simulink model "Simulation_Fahrmodell_v4_straight_line_v1"  (R2023b)
settings: Solver=ode14x  StartTime=0.0  StopTime=500  FixedStep=0.005  RelTol=1e-3
undefined symbols (not defined in the file): bat, cp, cp_Zelle_JpkgK, gb, Ice_derfacLoadDecrease_MAP, Ice_derfacLoadIncrease_MAP, Ice_n_axis, Ice_relLoadMax_CUR_n, Ice_relLoadMax_CUR_val, Ice_rl_axis_norm, P4, P4_DM, pt, seconds, SKO_STREET_CHAL, SKO_WHEEL_TYP_CHAL, slip_pacejka, T_init_degC, Track, TT_sliced, use_turbo_model, v_Fzg_init_kmph, veh
libraries: nesl_utility x15, fl_lib x9, simulink x4
(part 6 of 7)

== system Simulation_Fahrmodell_v4_straight_line_v1/Vehicle Dynamics Model /Drivetrain/Primary and Secondary Axle Powertrain Selector/Primary Axle Powertrain Selector/Electric Drive/Variant Subsystem/EV Single Motor/Battery and Operating Strategy Limitation (Drive)/Discharge Limit ==
  Torque_Drive_In : Inport
  Gain2 : Gain  Gain=100
  MATLAB Function : MATLAB Function  TreatAsAtomicUnit=on
  Recuperation Limit2 : Constant  Value=bat.SOC_Bat_Discharge_Limit
  Torque_Drive_Out : Outport
  wires:
  Torque_Drive_In/1 -> MATLAB Function/1(Torque_In)
  Recuperation Limit2/1 -> Gain2/1
  MATLAB Function/1(Torque_Out) -> Torque_Drive_Out/1
  [SOC] -> MATLAB Function/2(SOC)
  Gain2/1 -> MATLAB Function/3(Discharge_Limit)

== system Simulation_Fahrmodell_v4_straight_line_v1/Vehicle Dynamics Model /Drivetrain/Primary and Secondary Axle Powertrain Selector/Primary Axle Powertrain Selector/Electric Drive/Variant Subsystem/EV Single Motor/Battery and Operating Strategy Limitation (Recuperation)/Begrenzung BAT + Betriebsstrategie EM EV, Reku2 ==
  n_Upmin IN : Inport
  M_Nm : Inport  Port=2
  P_mech_max_kW : Inport  Port=3
  Max1 : MinMax  Function=max  Inputs=2
  "P_kW -> M_Nm" : Subsystem
  n_Upmin OUT : Outport
  M_begr_Nm : Outport  Port=2
  wires:
  M_Nm/1 -> Max1/1
  Max1/1 -> M_begr_Nm/1
  "P_kW -> M_Nm"/1(Out1) -> Max1/2  "M_mech_max_Nm"
  n_Upmin IN/1 -> "P_kW -> M_Nm"/2(In2), n_Upmin OUT/1
  P_mech_max_kW/1 -> "P_kW -> M_Nm"/1(P_kW)  "P_kW"

== system Simulation_Fahrmodell_v4_straight_line_v1/Vehicle Dynamics Model /Drivetrain/Primary and Secondary Axle Powertrain Selector/Primary Axle Powertrain Selector/Electric Drive/Variant Subsystem/EV Single Motor/Battery and Operating Strategy Limitation (Recuperation)/Recuperation Limit ==
  Torque_Recu_In : Inport
  Constant : Constant  Value=0
  Gain5 : Gain  Gain=100
  Recuperation Limit : Constant  Value=bat.SOC_Recup_Limit
  Relational Operator2 : RelationalOperator  Operator=<  OutDataTypeStr=boolean  RndMeth=Simplest  InputSameDT=off
  Switch2 : Switch  Criteria=u2 > Threshold  SaturateOnIntegerOverflow=off  InputSameDT=off
  Torque_Recu_Out : Outport
  wires:
  Constant/1 -> Switch2/3
  [SOC] -> Relational Operator2/1
  Recuperation Limit/1 -> Gain5/1
  Relational Operator2/1 -> Switch2/2
  Torque_Recu_In/1 -> Switch2/1
  Switch2/1 -> Torque_Recu_Out/1
  Gain5/1 -> Relational Operator2/2

== system Simulation_Fahrmodell_v4_straight_line_v1/Vehicle Dynamics Model /Drivetrain/Primary and Secondary Axle Powertrain Selector/Primary Axle Powertrain Selector/Hybrid Drive/P0/P0 Motor/Battery and Operating Strategy Limitation (Recuperation)/Begrenzung BAT + Betriebsstrategie EM P2, Reku1 ==
  n_Upmin IN : Inport
  M_Nm : Inport  Port=2
  P_mech_max_kW : Inport  Port=3
  Max1 : MinMax  Function=max  Inputs=2
  "P_kW -> M_Nm" : Subsystem
  n_Upmin OUT : Outport
  M_begr_Nm : Outport  Port=2
  wires:
  M_Nm/1 -> Max1/1
  Max1/1 -> M_begr_Nm/1
  "P_kW -> M_Nm"/1(Out1) -> Max1/2  "M_mech_max_Nm"
  n_Upmin IN/1 -> "P_kW -> M_Nm"/2(In2), n_Upmin OUT/1
  P_mech_max_kW/1 -> "P_kW -> M_Nm"/1(P_kW)  "P_kW"

== system Simulation_Fahrmodell_v4_straight_line_v1/Vehicle Dynamics Model /Drivetrain/Primary and Secondary Axle Powertrain Selector/Primary Axle Powertrain Selector/Hybrid Drive/P0/P0 Motor/Battery and Operating Strategy Limitation (Recuperation)/Recuperation Limit1 ==
  Torque_Recu_In : Inport
  Constant : Constant  Value=0
  Gain5 : Gain  Gain=100
  Recuperation Limit : Constant  Value=bat.SOC_Recup_Limit
  Relational Operator2 : RelationalOperator  Operator=<  OutDataTypeStr=boolean  RndMeth=Simplest  InputSameDT=off
  Switch2 : Switch  Criteria=u2 > Threshold  SaturateOnIntegerOverflow=off  InputSameDT=off
  Torque_Recu_Out : Outport
  wires:
  Constant/1 -> Switch2/3
  [SOC] -> Relational Operator2/1
  Recuperation Limit/1 -> Gain5/1
  Relational Operator2/1 -> Switch2/2
  Torque_Recu_In/1 -> Switch2/1
  Switch2/1 -> Torque_Recu_Out/1
  Gain5/1 -> Relational Operator2/2

== system Simulation_Fahrmodell_v4_straight_line_v1/Vehicle Dynamics Model /Drivetrain/Primary and Secondary Axle Powertrain Selector/Primary Axle Powertrain Selector/Hybrid Drive/P0/P0 Motor/SubsysteBattery and Operating Strategy Limitation (Drive)m/Begrenzung BAT + Betriebsstrategie EM P2, Fahren1 ==
  n_Upmin IN : Inport
  M_Nm : Inport  Port=2
  P_mech_max_kW : Inport  Port=3
  Max1 : MinMax  Inputs=2
  "P_kW -> M_Nm" : Subsystem
  n_Upmin OUT : Outport
  M_begr_Nm : Outport  Port=2
  wires:
  M_Nm/1 -> Max1/1
  Max1/1 -> M_begr_Nm/1
  "P_kW -> M_Nm"/1(Out1) -> Max1/2  "M_mech_max_Nm"
  n_Upmin IN/1 -> "P_kW -> M_Nm"/2(In2), n_Upmin OUT/1
  P_mech_max_kW/1 -> "P_kW -> M_Nm"/1(P_kW)  "P_kW"

== system Simulation_Fahrmodell_v4_straight_line_v1/Vehicle Dynamics Model /Drivetrain/Primary and Secondary Axle Powertrain Selector/Primary Axle Powertrain Selector/Hybrid Drive/P0/P0 Motor/SubsysteBattery and Operating Strategy Limitation (Drive)m/Discharge Limit ==
  Torque_Drive_In : Inport
  Gain2 : Gain  Gain=100
  MATLAB Function : MATLAB Function  TreatAsAtomicUnit=on
  Recuperation Limit2 : Constant  Value=bat.SOC_Bat_Discharge_Limit
  Torque_Drive_Out : Outport
  wires:
  Torque_Drive_In/1 -> MATLAB Function/1(Torque_In)
  Recuperation Limit2/1 -> Gain2/1
  MATLAB Function/1(Torque_Out) -> Torque_Drive_Out/1
  [SOC] -> MATLAB Function/2(SOC)
  Gain2/1 -> MATLAB Function/3(Discharge_Limit)

== system Simulation_Fahrmodell_v4_straight_line_v1/Vehicle Dynamics Model /Drivetrain/Primary and Secondary Axle Powertrain Selector/Primary Axle Powertrain Selector/Hybrid Drive/P2/P2 Motor/Battery and Operating Strategy Limitation (Drive)/Begrenzung BAT + Betriebsstrategie EM P2, Fahren1 ==
  n_Upmin IN : Inport
  M_Nm : Inport  Port=2
  P_mech_max_kW : Inport  Port=3
  Max1 : MinMax  Inputs=2
  "P_kW -> M_Nm" : Subsystem
  n_Upmin OUT : Outport
  M_begr_Nm : Outport  Port=2
  wires:
  M_Nm/1 -> Max1/1
  Max1/1 -> M_begr_Nm/1
  "P_kW -> M_Nm"/1(Out1) -> Max1/2  "M_mech_max_Nm"
  n_Upmin IN/1 -> "P_kW -> M_Nm"/2(In2), n_Upmin OUT/1
  P_mech_max_kW/1 -> "P_kW -> M_Nm"/1(P_kW)  "P_kW"

== system Simulation_Fahrmodell_v4_straight_line_v1/Vehicle Dynamics Model /Drivetrain/Primary and Secondary Axle Powertrain Selector/Primary Axle Powertrain Selector/Hybrid Drive/P2/P2 Motor/Battery and Operating Strategy Limitation (Drive)/Discharge Limit ==
  Torque_Drive_In : Inport
  Gain2 : Gain  Gain=100
  MATLAB Function : MATLAB Function  TreatAsAtomicUnit=on
  Recuperation Limit2 : Constant  Value=bat.SOC_Bat_Discharge_Limit
  Torque_Drive_Out : Outport
  wires:
  Torque_Drive_In/1 -> MATLAB Function/1(Torque_In)
  Recuperation Limit2/1 -> Gain2/1
  MATLAB Function/1(Torque_Out) -> Torque_Drive_Out/1
  [SOC] -> MATLAB Function/2(SOC)
  Gain2/1 -> MATLAB Function/3(Discharge_Limit)

== system Simulation_Fahrmodell_v4_straight_line_v1/Vehicle Dynamics Model /Drivetrain/Primary and Secondary Axle Powertrain Selector/Primary Axle Powertrain Selector/Hybrid Drive/P2/P2 Motor/Battery and Operating Strategy Limitation (Recuperation)/Begrenzung BAT + Betriebsstrategie EM P2, Reku1 ==
  n_Upmin IN : Inport
  M_Nm : Inport  Port=2
  P_mech_max_kW : Inport  Port=3
  Max1 : MinMax  Function=max  Inputs=2
  "P_kW -> M_Nm" : Subsystem
  n_Upmin OUT : Outport
  M_begr_Nm : Outport  Port=2
  wires:
  M_Nm/1 -> Max1/1
  Max1/1 -> M_begr_Nm/1
  "P_kW -> M_Nm"/1(Out1) -> Max1/2  "M_mech_max_Nm"
  n_Upmin IN/1 -> "P_kW -> M_Nm"/2(In2), n_Upmin OUT/1
  P_mech_max_kW/1 -> "P_kW -> M_Nm"/1(P_kW)  "P_kW"

== system Simulation_Fahrmodell_v4_straight_line_v1/Vehicle Dynamics Model /Drivetrain/Primary and Secondary Axle Powertrain Selector/Primary Axle Powertrain Selector/Hybrid Drive/P2/P2 Motor/Battery and Operating Strategy Limitation (Recuperation)/Recuperation Limit1 ==
  Torque_Recu_In : Inport
  Constant : Constant  Value=0
  Gain5 : Gain  Gain=100
  Recuperation Limit : Constant  Value=bat.SOC_Recup_Limit
  Relational Operator2 : RelationalOperator  Operator=<  OutDataTypeStr=boolean  RndMeth=Simplest  InputSameDT=off
  Switch2 : Switch  Criteria=u2 > Threshold  SaturateOnIntegerOverflow=off  InputSameDT=off
  Torque_Recu_Out : Outport
  wires:
  Constant/1 -> Switch2/3
  [SOC] -> Relational Operator2/1
  Recuperation Limit/1 -> Gain5/1
  Relational Operator2/1 -> Switch2/2
  Torque_Recu_In/1 -> Switch2/1
  Switch2/1 -> Torque_Recu_Out/1
  Gain5/1 -> Relational Operator2/2

== system Simulation_Fahrmodell_v4_straight_line_v1/Vehicle Dynamics Model /Drivetrain/Primary and Secondary Axle Powertrain Selector/Primary Axle Powertrain Selector/Hybrid Drive/P3/P3 Motor/Battery and Operating Strategy Limitation (Drive)/Begrenzung BAT + Betriebsstrategie EM P2, Fahren1 ==
  n_Upmin IN : Inport
  M_Nm : Inport  Port=2
  P_max_EM_kW : Inport  Port=3
  Max1 : MinMax  Inputs=2
  "P_kW -> M_Nm" : Subsystem
  n_Upmin OUT : Outport
  tq_sh_P3_bat_limted : Outport  Port=2
  wires:
  M_Nm/1 -> Max1/1
  Max1/1 -> tq_sh_P3_bat_limted/1
  "P_kW -> M_Nm"/1(Out1) -> Max1/2  "M_max_EM_Nm"
  n_Upmin IN/1 -> "P_kW -> M_Nm"/2(In2), n_Upmin OUT/1
  P_max_EM_kW/1 -> "P_kW -> M_Nm"/1(P_kW)  "P_kW"

== system Simulation_Fahrmodell_v4_straight_line_v1/Vehicle Dynamics Model /Drivetrain/Primary and Secondary Axle Powertrain Selector/Primary Axle Powertrain Selector/Hybrid Drive/P3/P3 Motor/Battery and Operating Strategy Limitation (Drive)/Discharge Limit ==
  Torque_Drive_In : Inport
  Add : Sum  Commented=on
  Constant : Constant  Commented=on  Value=0
  Constant1 : Constant  Commented=on  Value=10
  From1 : From  Commented=on  GotoTag=SOC  TagVisibility=global
  From8 : From  Commented=on  GotoTag=SOC  TagVisibility=global
  Gain1 : Gain  Commented=on  Gain=100
  Gain2 : Gain  Gain=100
  Gain5 : Gain  Commented=on  Gain=100
  MATLAB Function : MATLAB Function  TreatAsAtomicUnit=on
  Recuperation Limit : Constant  Commented=on  Value=bat.SOC_Bat_Discharge_Limit
  Recuperation Limit1 : Constant  Commented=on  Value=bat.SOC_Bat_Discharge_Limit
  Recuperation Limit2 : Constant  Value=bat.SOC_Bat_Discharge_Limit
  Relational Operator1 : RelationalOperator  Commented=on  Operator=>  OutDataTypeStr=boolean  RndMeth=Simplest  InputSameDT=off
  Relational Operator2 : RelationalOperator  Commented=on  Operator=>  OutDataTypeStr=boolean  RndMeth=Simplest  InputSameDT=off
  Switch1 : Switch  Commented=on  Criteria=u2 > Threshold  SaturateOnIntegerOverflow=off  InputSameDT=off
  Switch2 : Switch  Commented=on  Criteria=u2 > Threshold  SaturateOnIntegerOverflow=off  InputSameDT=off
  Torque_Drive_Out : Outport
  wires:
  Switch1/1 -> ?
  Recuperation Limit1/1 -> Gain1/1
  Add/1 -> Relational Operator1/2
  Relational Operator1/1 -> Switch1/2
  From1/1 -> Relational Operator1/1
  Gain1/1 -> Add/1
  Switch2/1 -> Switch1/1
  ? -> Switch2/1
  Recuperation Limit/1 -> Gain5/1
  Constant/1 -> Switch2/3, Switch1/3
  From8/1 -> Relational Operator2/1
  Relational Operator2/1 -> Switch2/2
  Constant1/1 -> Add/2
  Gain5/1 -> Relational Operator2/2
  Torque_Drive_In/1 -> MATLAB Function/1(Torque_In)
  Recuperation Limit2/1 -> Gain2/1
  MATLAB Function/1(Torque_Out) -> Torque_Drive_Out/1
  [SOC] -> MATLAB Function/2(SOC)
  Gain2/1 -> MATLAB Function/3(Discharge_Limit)

== system Simulation_Fahrmodell_v4_straight_line_v1/Vehicle Dynamics Model /Drivetrain/Primary and Secondary Axle Powertrain Selector/Primary Axle Powertrain Selector/Hybrid Drive/P3/P3 Motor/Battery and Operating Strategy Limitation (Recuperation)/Begrenzung BAT + Betriebsstrategie EM P2, Reku1 ==
  n_Upmin IN : Inport
  M_Nm : Inport  Port=2
  P_mech_max_kW : Inport  Port=3
  Max1 : MinMax  Function=max  Inputs=2
  "P_kW -> M_Nm" : Subsystem
  n_Upmin OUT : Outport
  M_begr_Nm : Outport  Port=2
  wires:
  M_Nm/1 -> Max1/1
  Max1/1 -> M_begr_Nm/1
  "P_kW -> M_Nm"/1(Out1) -> Max1/2  "M_mech_max_Nm"
  n_Upmin IN/1 -> "P_kW -> M_Nm"/2(In2), n_Upmin OUT/1
  P_mech_max_kW/1 -> "P_kW -> M_Nm"/1(P_kW)  "P_kW"

== system Simulation_Fahrmodell_v4_straight_line_v1/Vehicle Dynamics Model /Drivetrain/Primary and Secondary Axle Powertrain Selector/Primary Axle Powertrain Selector/Hybrid Drive/P3/P3 Motor/Battery and Operating Strategy Limitation (Recuperation)/Recuperation Limit1 ==
  Torque_Recu_In : Inport
  Constant : Constant  Value=0
  Gain5 : Gain  Gain=100
  Recuperation Limit : Constant  Value=bat.SOC_Recup_Limit
  Relational Operator2 : RelationalOperator  Operator=<  OutDataTypeStr=boolean  RndMeth=Simplest  InputSameDT=off
  Switch2 : Switch  Criteria=u2 > Threshold  SaturateOnIntegerOverflow=off  InputSameDT=off
  Torque_Recu_Out : Outport
  wires:
  Constant/1 -> Switch2/3
  [SOC] -> Relational Operator2/1
  Recuperation Limit/1 -> Gain5/1
  Relational Operator2/1 -> Switch2/2
  Torque_Recu_In/1 -> Switch2/1
  Switch2/1 -> Torque_Recu_Out/1
  Gain5/1 -> Relational Operator2/2

== system Simulation_Fahrmodell_v4_straight_line_v1/Vehicle Dynamics Model /Drivetrain/Primary and Secondary Axle Powertrain Selector/Secondary Axle Powertrain Selector/Auswahl P4, P4_Dual-Motor/P4 // E2 Single Motor/Battery and Operating Strategy Limitation (Drive)/Begrenzung BAT + Betriebsstrategie EM P4, Fahren1/P_kW -> M_Nm ==
  P_kW : Inport
  In2 : Inport  Port=2
  Constant : Constant
  Constant1 : Constant  Value=2*pi/60/1000
  Divide : Product  Inputs=*//
  Max2 : MinMax  Function=max  Inputs=2
  Out1 : Outport
  wires:
  Divide/1 -> Out1/1
  In2/1 -> Max2/1
  P_kW/1 -> Divide/1
  Constant1/1 -> Divide/2
  Max2/1 -> Divide/3
  Constant/1 -> Max2/2

== system Simulation_Fahrmodell_v4_straight_line_v1/Vehicle Dynamics Model /Drivetrain/Primary and Secondary Axle Powertrain Selector/Secondary Axle Powertrain Selector/Auswahl P4, P4_Dual-Motor/P4 // E2 Single Motor/Battery and Operating Strategy Limitation (Recuperation)/Begrenzung BAT + Betriebsstrategie EM P4, Reku1/P_kW -> M_Nm ==
  P_kW : Inport
  In2 : Inport  Port=2
  Constant : Constant
  Constant1 : Constant  Value=2*pi/60/1000
  Divide : Product  Inputs=*//
  Max2 : MinMax  Function=max  Inputs=2
  Out1 : Outport
  wires:
  Divide/1 -> Out1/1
  In2/1 -> Max2/1
  P_kW/1 -> Divide/1
  Constant1/1 -> Divide/2
  Max2/1 -> Divide/3
  Constant/1 -> Max2/2

== system Simulation_Fahrmodell_v4_straight_line_v1/Vehicle Dynamics Model /Drivetrain/Primary and Secondary Axle Powertrain Selector/Secondary Axle Powertrain Selector/Auswahl P4, P4_Dual-Motor/P4 // E3 // E4 Dual Motor/Battery and Operating Strategy Limitation (Drive) 1/Begrenzung BAT + Betriebsstrategie EM P4_DM_L, Fahren1/P_kW -> M_Nm ==
  P_kW : Inport
  In2 : Inport  Port=2
  Constant : Constant
  Constant1 : Constant  Value=2*pi/60/1000
  Divide : Product  Inputs=*//
  Max2 : MinMax  Function=max  Inputs=2
  Out1 : Outport
  wires:
  Divide/1 -> Out1/1
  In2/1 -> Max2/1
  P_kW/1 -> Divide/1
  Constant1/1 -> Divide/2
  Max2/1 -> Divide/3
  Constant/1 -> Max2/2

== system Simulation_Fahrmodell_v4_straight_line_v1/Vehicle Dynamics Model /Drivetrain/Primary and Secondary Axle Powertrain Selector/Secondary Axle Powertrain Selector/Auswahl P4, P4_Dual-Motor/P4 // E3 // E4 Dual Motor/Battery and Operating Strategy Limitation (Drive) 2/Begrenzung BAT + Betriebsstrategie EM P4_DM_R, Fahren2/P_kW -> M_Nm ==
  P_kW : Inport
  In2 : Inport  Port=2
  Constant : Constant
  Constant1 : Constant  Value=2*pi/60/1000
  Divide : Product  Inputs=*//
  Max2 : MinMax  Function=max  Inputs=2
  Out1 : Outport
  wires:
  Divide/1 -> Out1/1
  In2/1 -> Max2/1
  P_kW/1 -> Divide/1
  Constant1/1 -> Divide/2
  Max2/1 -> Divide/3
  Constant/1 -> Max2/2

== system Simulation_Fahrmodell_v4_straight_line_v1/Vehicle Dynamics Model /Drivetrain/Primary and Secondary Axle Powertrain Selector/Secondary Axle Powertrain Selector/Auswahl P4, P4_Dual-Motor/P4 // E3 // E4 Dual Motor/Battery and Operating Strategy Limitation (Recuperation) 1/Begrenzung BAT + Betriebsstrategie EM P4_DM_L, Reku1/P_kW -> M_Nm ==
  P_kW : Inport
  In2 : Inport  Port=2
  Constant : Constant
  Constant1 : Constant  Value=2*pi/60/1000
  Divide : Product  Inputs=*//
  Max2 : MinMax  Function=max  Inputs=2
  Out1 : Outport
  wires:
  Divide/1 -> Out1/1
  In2/1 -> Max2/1
  P_kW/1 -> Divide/1
  Constant1/1 -> Divide/2
  Max2/1 -> Divide/3
  Constant/1 -> Max2/2

== system Simulation_Fahrmodell_v4_straight_line_v1/Vehicle Dynamics Model /Drivetrain/Primary and Secondary Axle Powertrain Selector/Secondary Axle Powertrain Selector/Auswahl P4, P4_Dual-Motor/P4 // E3 // E4 Dual Motor/Battery and Operating Strategy Limitation (Recuperation) 2/Begrenzung BAT + Betriebsstrategie EM P4_DM_R, Reku2/P_kW -> M_Nm ==
  P_kW : Inport
  In2 : Inport  Port=2
  Constant : Constant
  Constant1 : Constant  Value=2*pi/60/1000
  Divide : Product  Inputs=*//
  Max2 : MinMax  Function=max  Inputs=2
  Out1 : Outport
  wires:
  Divide/1 -> Out1/1
  In2/1 -> Max2/1
  P_kW/1 -> Divide/1
  Constant1/1 -> Divide/2
  Max2/1 -> Divide/3
  Constant/1 -> Max2/2

== system Simulation_Fahrmodell_v4_straight_line_v1/Vehicle Dynamics Model /Drivetrain/Primary and Secondary Axle Powertrain Selector/Primary Axle Powertrain Selector/Electric Drive/Variant Subsystem/EV Dual Motor/Battery and Operating Strategy Limitation (Drive)/Begrenzung BAT + Betriebsstrategie EM P4_DM_L, Fahren2/P_kW -> M_Nm ==
  P_kW : Inport
  In2 : Inport  Port=2
  Constant : Constant
  Constant1 : Constant  Value=2*pi/60/1000
  Divide : Product  Inputs=*//
  Max2 : MinMax  Function=max  Inputs=2
  Out1 : Outport
  wires:
  Divide/1 -> Out1/1
  In2/1 -> Max2/1
  P_kW/1 -> Divide/1
  Constant1/1 -> Divide/2
  Max2/1 -> Divide/3
  Constant/1 -> Max2/2

== system Simulation_Fahrmodell_v4_straight_line_v1/Vehicle Dynamics Model /Drivetrain/Primary and Secondary Axle Powertrain Selector/Primary Axle Powertrain Selector/Electric Drive/Variant Subsystem/EV Dual Motor/Battery and Operating Strategy Limitation (Drive) /Begrenzung BAT + Betriebsstrategie EM P4_DM_R, Fahren1/P_kW -> M_Nm ==
  P_kW : Inport
  In2 : Inport  Port=2
  Constant : Constant
  Constant1 : Constant  Value=2*pi/60/1000
  Divide : Product  Inputs=*//
  Max2 : MinMax  Function=max  Inputs=2
  Out1 : Outport
  wires:
  Divide/1 -> Out1/1
  In2/1 -> Max2/1
  P_kW/1 -> Divide/1
  Constant1/1 -> Divide/2
  Max2/1 -> Divide/3
  Constant/1 -> Max2/2

== system Simulation_Fahrmodell_v4_straight_line_v1/Vehicle Dynamics Model /Drivetrain/Primary and Secondary Axle Powertrain Selector/Primary Axle Powertrain Selector/Electric Drive/Variant Subsystem/EV Dual Motor/Battery and Operating Strategy Limitation (Recuperation)/Begrenzung BAT + Betriebsstrategie EM P4_DM_L, Reku2/P_kW -> M_Nm ==
  P_kW : Inport
  In2 : Inport  Port=2
  Constant : Constant
  Constant1 : Constant  Value=2*pi/60/1000
  Divide : Product  Inputs=*//
  Max2 : MinMax  Function=max  Inputs=2
  Out1 : Outport
  wires:
  Divide/1 -> Out1/1
  In2/1 -> Max2/1
  P_kW/1 -> Divide/1
  Constant1/1 -> Divide/2
  Max2/1 -> Divide/3
  Constant/1 -> Max2/2

== system Simulation_Fahrmodell_v4_straight_line_v1/Vehicle Dynamics Model /Drivetrain/Primary and Secondary Axle Powertrain Selector/Primary Axle Powertrain Selector/Electric Drive/Variant Subsystem/EV Dual Motor/Battery and Operating Strategy Limitation (Recuperation) /Begrenzung BAT + Betriebsstrategie EM P4_DM_R, Reku1/P_kW -> M_Nm ==
  P_kW : Inport
  In2 : Inport  Port=2
  Constant : Constant
  Constant1 : Constant  Value=2*pi/60/1000
  Divide : Product  Inputs=*//
  Max2 : MinMax  Function=max  Inputs=2
  Out1 : Outport
  wires:
  Divide/1 -> Out1/1
  In2/1 -> Max2/1
  P_kW/1 -> Divide/1
  Constant1/1 -> Divide/2
  Max2/1 -> Divide/3
  Constant/1 -> Max2/2

== system Simulation_Fahrmodell_v4_straight_line_v1/Vehicle Dynamics Model /Drivetrain/Primary and Secondary Axle Powertrain Selector/Primary Axle Powertrain Selector/Electric Drive/Variant Subsystem/EV Single Motor/Battery and Operating Strategy Limitation (Drive)/Begrenzung BAT + Betriebsstrategie EM EV, Fahren2/P_kW -> M_Nm ==
  P_kW : Inport
  In2 : Inport  Port=2
  Constant : Constant
  Constant1 : Constant  Value=2*pi/60/1000
  Divide : Product  Inputs=*//
  Max2 : MinMax  Function=max  Inputs=2
  Out1 : Outport
  wires:
  Divide/1 -> Out1/1
  In2/1 -> Max2/1
  P_kW/1 -> Divide/1
  Constant1/1 -> Divide/2
  Max2/1 -> Divide/3
  Constant/1 -> Max2/2

== system Simulation_Fahrmodell_v4_straight_line_v1/Vehicle Dynamics Model /Drivetrain/Primary and Secondary Axle Powertrain Selector/Primary Axle Powertrain Selector/Electric Drive/Variant Subsystem/EV Single Motor/Battery and Operating Strategy Limitation (Recuperation)/Begrenzung BAT + Betriebsstrategie EM EV, Reku2/P_kW -> M_Nm ==
  P_kW : Inport
  In2 : Inport  Port=2
  Constant : Constant
  Constant1 : Constant  Value=2*pi/60/1000
  Divide : Product  Inputs=*//
  Max2 : MinMax  Function=max  Inputs=2
  Out1 : Outport
  wires:
  Divide/1 -> Out1/1
  In2/1 -> Max2/1
  P_kW/1 -> Divide/1
  Constant1/1 -> Divide/2
  Max2/1 -> Divide/3
  Constant/1 -> Max2/2

== system Simulation_Fahrmodell_v4_straight_line_v1/Vehicle Dynamics Model /Drivetrain/Primary and Secondary Axle Powertrain Selector/Primary Axle Powertrain Selector/Hybrid Drive/P0/P0 Motor/Battery and Operating Strategy Limitation (Recuperation)/Begrenzung BAT + Betriebsstrategie EM P2, Reku1/P_kW -> M_Nm ==
  P_kW : Inport
  In2 : Inport  Port=2
  Constant : Constant
  Constant1 : Constant  Value=2*pi/60/1000
  Divide : Product  Inputs=*//
  Max2 : MinMax  Function=max  Inputs=2
  Out1 : Outport
  wires:
  Divide/1 -> Out1/1
  In2/1 -> Max2/1
  P_kW/1 -> Divide/1
  Constant1/1 -> Divide/2
  Max2/1 -> Divide/3
  Constant/1 -> Max2/2

== system Simulation_Fahrmodell_v4_straight_line_v1/Vehicle Dynamics Model /Drivetrain/Primary and Secondary Axle Powertrain Selector/Primary Axle Powertrain Selector/Hybrid Drive/P0/P0 Motor/SubsysteBattery and Operating Strategy Limitation (Drive)m/Begrenzung BAT + Betriebsstrategie EM P2, Fahren1/P_kW -> M_Nm ==
  P_kW : Inport
  In2 : Inport  Port=2
  Constant : Constant
  Constant1 : Constant  Value=2*pi/60/1000
  Divide : Product  Inputs=*//
  Max2 : MinMax  Function=max  Inputs=2
  Out1 : Outport
  wires:
  Divide/1 -> Out1/1
  In2/1 -> Max2/1
  P_kW/1 -> Divide/1
  Constant1/1 -> Divide/2
  Max2/1 -> Divide/3
  Constant/1 -> Max2/2

== system Simulation_Fahrmodell_v4_straight_line_v1/Vehicle Dynamics Model /Drivetrain/Primary and Secondary Axle Powertrain Selector/Primary Axle Powertrain Selector/Hybrid Drive/P2/P2 Motor/Battery and Operating Strategy Limitation (Drive)/Begrenzung BAT + Betriebsstrategie EM P2, Fahren1/P_kW -> M_Nm ==
  P_kW : Inport
  In2 : Inport  Port=2
  Constant : Constant
  Constant1 : Constant  Value=2*pi/60/1000
  Divide : Product  Inputs=*//
  Max2 : MinMax  Function=max  Inputs=2
  Out1 : Outport
  wires:
  Divide/1 -> Out1/1
  In2/1 -> Max2/1
  P_kW/1 -> Divide/1
  Constant1/1 -> Divide/2
  Max2/1 -> Divide/3
  Constant/1 -> Max2/2

== system Simulation_Fahrmodell_v4_straight_line_v1/Vehicle Dynamics Model /Drivetrain/Primary and Secondary Axle Powertrain Selector/Primary Axle Powertrain Selector/Hybrid Drive/P2/P2 Motor/Battery and Operating Strategy Limitation (Recuperation)/Begrenzung BAT + Betriebsstrategie EM P2, Reku1/P_kW -> M_Nm ==
  P_kW : Inport
  In2 : Inport  Port=2
  Constant : Constant
  Constant1 : Constant  Value=2*pi/60/1000
  Divide : Product  Inputs=*//
  Max2 : MinMax  Function=max  Inputs=2
  Out1 : Outport
  wires:
  Divide/1 -> Out1/1
  In2/1 -> Max2/1
  P_kW/1 -> Divide/1
  Constant1/1 -> Divide/2
  Max2/1 -> Divide/3
  Constant/1 -> Max2/2

== system Simulation_Fahrmodell_v4_straight_line_v1/Vehicle Dynamics Model /Drivetrain/Primary and Secondary Axle Powertrain Selector/Primary Axle Powertrain Selector/Hybrid Drive/P3/P3 Motor/Battery and Operating Strategy Limitation (Drive)/Begrenzung BAT + Betriebsstrategie EM P2, Fahren1/P_kW -> M_Nm ==
  P_kW : Inport
  In2 : Inport  Port=2
  Constant : Constant
  Constant1 : Constant  Value=2*pi/60/1000
  Divide : Product  Inputs=*//
  Max2 : MinMax  Function=max  Inputs=2
  Out1 : Outport
  wires:
  Divide/1 -> Out1/1
  In2/1 -> Max2/1
  P_kW/1 -> Divide/1
  Constant1/1 -> Divide/2
  Max2/1 -> Divide/3
  Constant/1 -> Max2/2

== system Simulation_Fahrmodell_v4_straight_line_v1/Vehicle Dynamics Model /Drivetrain/Primary and Secondary Axle Powertrain Selector/Primary Axle Powertrain Selector/Hybrid Drive/P3/P3 Motor/Battery and Operating Strategy Limitation (Recuperation)/Begrenzung BAT + Betriebsstrategie EM P2, Reku1/P_kW -> M_Nm ==
  P_kW : Inport
  In2 : Inport  Port=2
  Constant : Constant
  Constant1 : Constant  Value=2*pi/60/1000
  Divide : Product  Inputs=*//
  Max2 : MinMax  Function=max  Inputs=2
  Out1 : Outport
  wires:
  Divide/1 -> Out1/1
  In2/1 -> Max2/1
  P_kW/1 -> Divide/1
  Constant1/1 -> Divide/2
  Max2/1 -> Divide/3
  Constant/1 -> Max2/2

== matlab function Simulation_Fahrmodell_v4_straight_line_v1/Vehicle Dynamics Model /Drivetrain/GETRIEBE auswahl VK, EV/Transmission Selector1/ICE Multi-Speed/Subsystem1/Shift Delay and Clutch Disengagement  ==
  settings: updateMethod=DISCRETE
  data: desiredGear input; currentGear output; dt input; clutchEngaged output; shiftDelay input
function [currentGear, clutchEngaged] = gearStep(desiredGear, dt, shiftDelay)
% Moves gear toward desiredGear one step at a time with a delay
% Also outputs clutchEngaged: 1 = engaged, 0 = disengaged

% shiftDelay = 0.3;   % seconds between shifts (tune this)

persistent gear timer shifting

if isempty(gear)
    gear = 1;
    timer = 0;
    shifting = false;
end

% Default: clutch engaged unless shifting
clutchEngaged = 1;

% If already at desired gear: no shift
if gear == desiredGear
    shifting = false;
    timer = 0;
    currentGear = gear;
    return;
end

% If not shifting yet, start shift timer
if ~shifting
    shifting = true;
    timer = 0;
end

% During shifting → clutch disengaged
clutchEngaged = 0;

% Accumulate time
timer = timer + dt;

% When delay elapsed, shift one step
if timer >= shiftDelay
    if desiredGear > gear
        gear = gear + 1;
    elseif desiredGear < gear
        gear = gear - 1;
    end

    timer = 0;

    % Stop shifting if reached target
    if gear == desiredGear
        shifting = false;
        clutchEngaged = 1;   % re-engage clutch immediately after shift
    end
end

currentGear = gear;

%% 2
% function currentGear = gearStep(desiredGear, dt)
% % Moves gear toward desiredGear one step at a time with a delay
% 
% shiftDelay = 1;   % seconds between shifts (tune this)
% 
% persistent gear timer shifting
% 
% if isempty(gear)
%     gear = 1;
%     timer = 0;
%     shifting = false;
% end
% 
% % If already at desired gear: no shift
% if gear == desiredGear
%     shifting = false;
%     timer = 0;
%     currentGear = gear;
%     return;
% end
% 
% % If not shifting yet, start shift timer
% if ~shifting
%     shifting = true;
%     timer = 0;
% end
% 
% % Accumulate time
% timer = timer + dt;
% 
% % When delay elapsed, shift one step
% if timer >= shiftDelay
%     if desiredGear > gear
%         gear = gear + 1;
%     elseif desiredGear < gear
%         gear = gear - 1;
%     end
% 
%     timer = 0;
% 
%     % Stop shifting if reached target
%     if gear == desiredGear
%         shifting = false;
%     end
% end
% 
% currentGear = gear;

== matlab function Simulation_Fahrmodell_v4_straight_line_v1/Vehicle Dynamics Model /Drivetrain/GETRIEBE auswahl VK, EV/Transmission Selector1/ICE Multi-Speed/Subsystem1/gear latch ==
  settings: updateMethod=DISCRETE
  data: upshift input; shift_cmd output; downshift input; cmd_Bypass_Lock_time input
function shift_cmd = gearLatch(upshift, downshift, cmd_Bypass_Lock_time)

persistent lockTimer
persistent pulseTimer
persistent lastDirection

LOCK_TIME  = 3.0;       % seconds
DT         = 0.005;     % timestep
PULSE_TIME = DT * 100;  % your working pulse duration

if isempty(lockTimer)
    lockTimer     = 0;
    pulseTimer    = 0;
    lastDirection = 0;
end

% Count down timers
lockTimer  = max(0, lockTimer - DT);
pulseTimer = max(0, pulseTimer - DT);

% Default output
shift_cmd = 0;

% If pulse is active, output last direction
if pulseTimer > 0
    shift_cmd = lastDirection;
    return
end

% Determine if lock should be bypassed
lockExpired = (lockTimer <= 0) || (cmd_Bypass_Lock_time == 1);

% Only allow shift when lock expired OR bypass active
if lockExpired

    % UPSHIFT
    if upshift && ~downshift
        lastDirection = 1;
        shift_cmd     = 1;
        pulseTimer    = PULSE_TIME;
        lockTimer     = LOCK_TIME;   % restart lock
        return
    end

    % DOWNSHIFT
    if downshift && ~upshift
        lastDirection = -1;
        shift_cmd     = -1;
        pulseTimer    = PULSE_TIME;
        lockTimer     = LOCK_TIME;   % restart lock
        return
    end
end
%% Current Final
% function shift_cmd = gearLatch(upshift, downshift)
% 
% persistent lockTimer
% persistent pulseTimer
% persistent lastDirection
% 
% LOCK_TIME  = 3.0;     % seconds
% DT         = 0.005;   % timestep
% PULSE_TIME = DT * 100;  % your working pulse duration
% 
% if isempty(lockTimer)
%     lockTimer     = 0;
%     pulseTimer    = 0;
%     lastDirection = 0;
% end
% 
% % Count down timers
% lockTimer  = max(0, lockTimer - DT);
% pulseTimer = max(0, pulseTimer - DT);
% 
% % Default output
% shift_cmd = 0;
% 
% % If pulse is active, output the last direction
% if pulseTimer > 0
%     shift_cmd = lastDirection;
%     return
% end
% 
% % Only allow new shift when lock expired
% if lockTimer <= 0
% 
%     % UPSHIFT
%     if upshift && ~downshift
%         lastDirection = 1;          % store direction
%         shift_cmd     = 1;
%         pulseTimer    = PULSE_TIME;
%         lockTimer     = LOCK_TIME;
%         return
%     end
% 
%     % DOWNSHIFT
%     if downshift && ~upshift
%         lastDirection = -1;         % store direction
%         shift_cmd     = -1;
%         pulseTimer    = PULSE_TIME;
%         lockTimer     = LOCK_TIME;
%         return
%     end
% end


% function shift_cmd = gearLatch(upshift, downshift)
% 
% persistent lastState lockTimer
% 
% LOCK_TIME = 3.0;   % seconds — post-shift hold (tune between 1.5–3.0)
% DT        = 0.005; % your fixed simulation timestep
% 
% if isempty(lastState)
%     lastState = 0;
%     lockTimer = 0;
% end
% 
% % Count down lockout
% lockTimer = max(0, lockTimer - DT);
% 
% % Only accept new command when lockout has expired
% if lockTimer <= 0
%     if upshift && ~downshift
%         if lastState ~= 1        % only trigger on direction change
%             lastState = 1;
%             lockTimer = LOCK_TIME;
%         end
%     elseif downshift && ~upshift
%         if lastState ~= -1
%             lastState = -1;
%             lockTimer = LOCK_TIME;
%         end
%     else
%         lastState = 0;           % no command active → clear latch
%     end
% end
% 
% shift_cmd = lastState;
%% 
% function shift_cmd = gearLatch(upshift, downshift)
% 
% % gearLatch: Latches shift direction until opposite condition occurs
% % Persistent variable to store last state
% % 1 = upshift latched
% % -1 = downshift latched
% % 0 = no shift
% persistent lastState
% if isempty(lastState)
%     lastState = 0;
% end
% % Update latch
% if upshift
%     lastState = 1;
% elseif downshift
%     lastState = -1;
% elseif ~upshift && ~downshift
%     lastState = 0;
% end
% 
% % Output the latched state
% shift_cmd = lastState;


%% 3 sec

% function shift_cmd = gearLatch(upshift, downshift, t, lockout_time)
% % gearLatch: Latches shift direction and enforces a time lockout to prevent hunting.
% % Inputs:
% %   upshift      - Boolean upshift command
% %   downshift    - Boolean downshift command
% %   t            - Current time (seconds)
% %   lockout_time - Minimum time required between shifts (seconds)
% 
% persistent lastState lastShiftTime
% 
% % Initialize persistent variables on first pass
% if isempty(lastState)
%     lastState = 0;
%     lastShiftTime = -inf; % Ensure we can shift immediately at start
% end
% 
% % Evaluate shift commands ONLY if the lockout period has expired
% if (t - lastShiftTime) > lockout_time
%     if upshift
%         lastState = 1;
%         lastShiftTime = t; % Reset timer
%     elseif downshift
%         lastState = -1;
%         lastShiftTime = t; % Reset timer
%     else
%         lastState = 0; % Optional: Reset to neutral/steady state if needed
%     end
% end
% 
% % Output the latched state
% shift_cmd = lastState;

== matlab function Simulation_Fahrmodell_v4_straight_line_v1/Vehicle Dynamics Model /Drivetrain/GETRIEBE auswahl VK, EV/Transmission Selector/ICE Multi-Speed/MATLAB Function ==
  data: gearOld output; gearTarget output; n_current input; gearActual output; n_min_in input; n_max_in input; shiftDelay input; dt input; nGears input; shiftAlpha output
function [gearOld, gearTarget, gearActual, shiftAlpha] = ShiftManagerRatioBlend( ...
    n_current, n_min_in, n_max_in, shiftDelay, dt, nGears)

persistent gear oldGear targetGear timer shifting holdTimer

if isempty(gear)
    gear = 1;
    oldGear = 1;
    targetGear = 1;
    timer = 0;
    shifting = false;
    holdTimer = 0;
end

% Safety
if nGears < 1
    nGears = 1;
end

gear = min(max(gear, 1), nGears);

% Robust gegen vertauschte Eingänge
n_min = min(n_min_in, n_max_in); %#ok<NASGU>
n_max = max(n_min_in, n_max_in);

% Default
shiftAlpha = 1;

% Ein-Gang-System
if nGears <= 1
    gear = 1;
    oldGear = 1;
    targetGear = 1;
    timer = 0;
    shifting = false;
    holdTimer = 0;

    gearOld = 1;
    gearTarget = 1;
    gearActual = 1;
    shiftAlpha = 1;
    return;
end

% kurze Sperrzeit nach abgeschlossener Schaltung
if holdTimer > 0
    holdTimer = holdTimer - dt;
end

% Nur Hochschalten für 0-100 Vollgas
if ~shifting && holdTimer <= 0

    if n_current >= n_max && gear < nGears
        oldGear = gear;
        targetGear = gear + 1;
        timer = 0;
        shifting = true;
    end
end

% Während Schaltung: alpha von 0 auf 1
if shifting

    timer = timer + dt;

    if shiftDelay <= 0
        shiftAlpha = 1;
    else
        shiftAlpha = timer / shiftDelay;
    end

    shiftAlpha = min(max(shiftAlpha, 0), 1);

    if shiftAlpha >= 1
        gear = targetGear;
        oldGear = gear;
        shifting = false;
        timer = 0;
        shiftAlpha = 1;

        % verhindert sofortiges Weiterschalten durch i_GES_delay
        holdTimer = max(0.05, 2 * dt);
    end

else
    oldGear = gear;
    targetGear = gear;
    shiftAlpha = 1;
end

gearOld = oldGear;
gearTarget = targetGear;
gearActual = gear;

== matlab function Simulation_Fahrmodell_v4_straight_line_v1/Vehicle Dynamics Model /Drivetrain/GETRIEBE auswahl VK, EV/Transmission Selector/ICE Multi-Speed/Weicher Übergang ==
  data: i_old input; i_eff output; i_target input; alpha input
function i_eff = BlendRatio(i_old, i_target, alpha)

% alpha begrenzen
if alpha < 0
    alpha = 0;
elseif alpha > 1
    alpha = 1;
end

% weicher Verlauf 0 -> 1
s = alpha * alpha * (3 - 2 * alpha);

% Übersetzung überblenden
i_eff = (1 - s) * i_old + s * i_target;

== matlab function Simulation_Fahrmodell_v4_straight_line_v1/Vehicle Dynamics Model /Drivetrain/Axle Load and Torque Distribution /Berechnung Achslastverteilung abh. Fahrzeugeigenschaften (Haken Abs. 11)/MATLAB Function ==
  data: u input; y output
function y = cosd(u)

y = cosd(u);

== matlab function Simulation_Fahrmodell_v4_straight_line_v1/Vehicle Dynamics Model /Drivetrain/Axle Load and Torque Distribution /Berechnung Achslastverteilung abh. Fahrzeugeigenschaften (Haken Abs. 11)/MATLAB Function1 ==
  data: u input; y output
function y = sind(u)

y = sind(u);

== matlab function Simulation_Fahrmodell_v4_straight_line_v1/Vehicle Dynamics Model /Drivetrain/Axle Load and Torque Distribution /MATLAB Function ==
  data: Tq_Primary input; Tq_FrontAxle output; Tq_Secondary input; HM_VA input; AWD input; P4 input; P4_DM input; MainSplit input; Tq_RearAxle output; Tq_grip_FrontMax input; Tq_grip_RearMax input
function [Tq_FrontAxle, Tq_RearAxle] = routeAxleTorqueDynamic( ...
    Tq_Primary, Tq_Secondary, HM_VA, AWD, P4, P4_DM, MainSplit, ...
    Tq_grip_FrontMax, Tq_grip_RearMax)

hasP4 = (P4 == 1) || (P4_DM == 1);

Tq_FrontAxle = 0;
Tq_RearAxle  = 0;

if MainSplit < 0
    MainSplit = 0;
elseif MainSplit > 1
    MainSplit = 1;
end

if AWD == 1 && ~hasP4
    % Mechanisches / variables AWD ohne P4:
    % Gesamtmoment dynamisch nach verfügbarer Traktion verteilen.

    Tq_total = max(Tq_Primary, 0) + max(Tq_Secondary, 0);

    capFront = max(Tq_grip_FrontMax, 0);
    capRear  = max(Tq_grip_RearMax, 0);
    capSum   = capFront + capRear;

    if capSum > 1e-6
        frontShare = capFront / capSum;
    else
        % Fallback: statischer Split
        if HM_VA == 1
            frontShare = MainSplit;
        else
            frontShare = 1 - MainSplit;
        end
    end

    % Optional: nicht zu extreme Splits erlauben
    if frontShare < 0.25
        frontShare = 0.25;
    elseif frontShare > 0.75
        frontShare = 0.75;
    end

    Tq_FrontAxle = frontShare * Tq_total;
    Tq_RearAxle  = (1 - frontShare) * Tq_total;

elseif hasP4
    % P4-Fall: Primary und Secondary bleiben separate Achsantriebe.
    if HM_VA == 1
        Tq_FrontAxle = Tq_Primary;
        Tq_RearAxle  = Tq_Secondary;
    else
        Tq_RearAxle  = Tq_Primary;
        Tq_FrontAxle = Tq_Secondary;
    end

else
    % 2WD-Fall
    if HM_VA == 1
        Tq_FrontAxle = Tq_Primary;
        Tq_RearAxle  = 0;
    else
        Tq_RearAxle  = Tq_Primary;
        Tq_FrontAxle = 0;
    end
end
end

== matlab function Simulation_Fahrmodell_v4_straight_line_v1/Vehicle Dynamics Model /Drivetrain/Operating Strategy 1.1/Axle Torque Split/MATLAB Function1 ==
  data: P4_deactivate output; Torque_ICE_Axle_percent output; SOC input; cfg_P4 input; EV input; MainAxle_TorqueSplit_int input; Torque_P4_Axle_percent output
function [P4_deactivate, Torque_ICE_Axle_percent, Torque_P4_Axle_percent]...
        = TorqueSplit(SOC, cfg_P4, EV, MainAxle_TorqueSplit_int)

    % State memory for hysteresis (Lockout flag)
    persistent p4_low_soc_lockout
    if isempty(p4_low_soc_lockout)
        p4_low_soc_lockout = false; 
    end

    % Default: ICE takes all torque, P4 takes none
    Torque_ICE_Axle_percent = 1;
    Torque_P4_Axle_percent = 0;
    P4_deactivate = 0;

    if EV == 1
        P4_split = 1 - MainAxle_TorqueSplit_int;
        Torque_P4_Axle_percent = P4_split;
        Torque_ICE_Axle_percent = 1 - P4_split;
        
    elseif cfg_P4 == 1
        % User-defined P4 split (Main axle = ICE)
        P4_split = 1 - MainAxle_TorqueSplit_int;

        % --- HYSTERESIS LOGIC START ---
        % 1. Determine Lockout State
        if SOC < 0.20
            p4_low_soc_lockout = true;       % Drop below 20%: Lock P4
        elseif SOC >= 0.25
            p4_low_soc_lockout = false;      % Rise above 25%: Unlock P4
        end

        % 2. Apply Limits based on State & SOC
        if p4_low_soc_lockout
            P4_limit = 0;                    % Locked state: 0 torque
        elseif SOC < 0.5
            P4_limit = 0.20;                 % Unlocked but low SOC: Limited torque
        else
            P4_limit = P4_split;             % Healthy SOC: No restriction
        end
        % --- HYSTERESIS LOGIC END ---

        % Apply restriction only if user-defined split exceeds limit
        P4_split = min(P4_split, P4_limit);

        if P4_split == 0
            P4_deactivate = 1;
        else
            P4_deactivate = 0;
        end

        % Assign outputs
        Torque_P4_Axle_percent = P4_split;
        Torque_ICE_Axle_percent = 1 - P4_split;
    end
end

== matlab function Simulation_Fahrmodell_v4_straight_line_v1/Vehicle Dynamics Model /Drivetrain/Operating Strategy 1.1/EM Torque Distributor ==
  data: tq_wheel_EL_des input; tq_wheel_P0_des output; tq_wheel_P2_des output; tq_wheel_P3_des output; Pwr_P0_max_kW input; Pwr_P2_max_kW input; Pwr_P3_max_kW input; cfg_P0 input; cfg_P2 input; cfg_P3 input
function [tq_wheel_P0_des, tq_wheel_P2_des, tq_wheel_P3_des] = ...
    TorqueSplit(tq_wheel_EL_des, Pwr_P0_max_kW, Pwr_P2_max_kW, Pwr_P3_max_kW, ...
                cfg_P0, cfg_P2, cfg_P3)

    % Apply configuration: if cfg = 0, power = 0 (machine disabled)
    P0_active = Pwr_P0_max_kW * cfg_P0;
    P2_active = Pwr_P2_max_kW * cfg_P2;
    P3_active = Pwr_P3_max_kW * cfg_P3;
    
    % Total available power from active machines
    totalPwr = P0_active + P2_active + P3_active;

    % Avoid division by zero (no machine active)
    if totalPwr == 0
        tq_wheel_P0_des = 0;
        tq_wheel_P2_des = 0;
        tq_wheel_P3_des = 0;
        return
    end

    % Ratios based only on active machines
    ratio_P0 = P0_active / totalPwr;
    ratio_P2 = P2_active / totalPwr;
    ratio_P3 = P3_active / totalPwr;

    % Torque split
    tq_wheel_P0_des = ratio_P0 * tq_wheel_EL_des;
    tq_wheel_P2_des = ratio_P2 * tq_wheel_EL_des;
    tq_wheel_P3_des = ratio_P3 * tq_wheel_EL_des;

end

== matlab function Simulation_Fahrmodell_v4_straight_line_v1/Vehicle Dynamics Model /Drivetrain/Operating Strategy 1.1/EMs Priority (Ep)/MATLAB Function ==
  data: tq_ICE_in input; tq_ICE_out output; tq_Elec_in input; SOC input; tq_Elec_out output
function [tq_ICE_out, tq_Elec_out] = TorqueReallocation(tq_ICE_in, tq_Elec_in, SOC)

    % -------------------------------------------------------------
    % HYSTERESIS STATE MEMORY
    % -------------------------------------------------------------
    persistent elec_blocked
    if isempty(elec_blocked)
        elec_blocked = false; % Default: Electric enabled
    end

    % Thresholds
    SOC_Limit = 20;               % Cutoff limit (from your Green block)
    Recovery_Threshold = 25;      % Limit + 5% Hysteresis

    % -------------------------------------------------------------
    % UPDATE STATE (The "Delay Thing")
    % -------------------------------------------------------------
    if SOC < SOC_Limit
        elec_blocked = true;      % SOC dropped too low -> Block Elec
    elseif SOC >= Recovery_Threshold
        elec_blocked = false;     % SOC recovered enough -> Restore Elec
    end
    % Note: If SOC is between 20 and 25, 'elec_blocked' keeps its previous value

    % -------------------------------------------------------------
    % TORQUE LOGIC (From your Diagram)
    % -------------------------------------------------------------
    if elec_blocked
        % LOGIC: SOC is Low (Switch F position)
        % Electric is zeroed.
        % Electric demand is shifted (added) to ICE to compensate.
        tq_Elec_out = 0;
        tq_ICE_out  = tq_ICE_in + tq_Elec_in;
        
    else
        % LOGIC: SOC is Healthy (Switch T position)
        % Inputs pass through unchanged.
        tq_Elec_out = tq_Elec_in;
        tq_ICE_out  = tq_ICE_in;
    end

end

== matlab function Simulation_Fahrmodell_v4_straight_line_v1/Vehicle Dynamics Model /Drivetrain/Primary and Secondary Axle Powertrain Selector/Primary Axle Powertrain Selector/Electric Drive/Variant Subsystem/EV Dual Motor/Battery and Operating Strategy Limitation (Drive)/Discharge Limit/MATLAB Function ==
  settings: updateMethod=DISCRETE
  data: Torque_In input; SOC input; Torque_Out output; Discharge_Limit input
function Torque_Out = fcn(Torque_In, SOC, Discharge_Limit)

% -------------------------------------------------------------
% Corrected SOC Hysteresis Logic
% -------------------------------------------------------------
% If SOC < Discharge_Limit → torque blocked
% Torque stays blocked until SOC >= Discharge_Limit + 10
% -------------------------------------------------------------

persistent torque_blocked

if isempty(torque_blocked)
    torque_blocked = false;   % Start with torque allowed
end

% Hysteresis threshold
Recovery_Threshold = Discharge_Limit + 5;

% --- BLOCKING CONDITION --------------------------------------
if SOC < Discharge_Limit
    torque_blocked = true;
end

% --- RECOVERY CONDITION --------------------------------------
if torque_blocked
    if SOC >= Recovery_Threshold
        torque_blocked = false;   % SOC recovered enough
    else
        Torque_Out = 0;           % Still blocked
        return
    end
end

% --- NORMAL OPERATION ----------------------------------------
Torque_Out = Torque_In;

end

== matlab function Simulation_Fahrmodell_v4_straight_line_v1/Vehicle Dynamics Model /Drivetrain/Primary and Secondary Axle Powertrain Selector/Primary Axle Powertrain Selector/Electric Drive/Variant Subsystem/EV Dual Motor/Battery and Operating Strategy Limitation (Drive) /Discharge Limit1/MATLAB Function ==
  settings: updateMethod=DISCRETE
  data: Torque_In input; SOC input; Torque_Out output; Discharge_Limit input
function Torque_Out = fcn(Torque_In, SOC, Discharge_Limit)

% -------------------------------------------------------------
% Corrected SOC Hysteresis Logic
% -------------------------------------------------------------
% If SOC < Discharge_Limit → torque blocked
% Torque stays blocked until SOC >= Discharge_Limit + 10
% -------------------------------------------------------------

persistent torque_blocked

if isempty(torque_blocked)
    torque_blocked = false;   % Start with torque allowed
end

% Hysteresis threshold
Recovery_Threshold = Discharge_Limit + 5;

% --- BLOCKING CONDITION --------------------------------------
if SOC < Discharge_Limit
    torque_blocked = true;
end

% --- RECOVERY CONDITION --------------------------------------
if torque_blocked
    if SOC >= Recovery_Threshold
        torque_blocked = false;   % SOC recovered enough
    else
        Torque_Out = 0;           % Still blocked
        return
    end
end

% --- NORMAL OPERATION ----------------------------------------
Torque_Out = Torque_In;

end

== matlab function Simulation_Fahrmodell_v4_straight_line_v1/Vehicle Dynamics Model /Drivetrain/Primary and Secondary Axle Powertrain Selector/Primary Axle Powertrain Selector/Electric Drive/Variant Subsystem/EV Single Motor/Battery and Operating Strategy Limitation (Drive)/Discharge Limit/MATLAB Function ==
  settings: updateMethod=DISCRETE
  data: Torque_In input; SOC input; Torque_Out output; Discharge_Limit input
function Torque_Out = fcn(Torque_In, SOC, Discharge_Limit)

% -------------------------------------------------------------
% Corrected SOC Hysteresis Logic
% -------------------------------------------------------------
% If SOC < Discharge_Limit → torque blocked
% Torque stays blocked until SOC >= Discharge_Limit + 10
% -------------------------------------------------------------

persistent torque_blocked

if isempty(torque_blocked)
    torque_blocked = false;   % Start with torque allowed
end

% Hysteresis threshold
Recovery_Threshold = Discharge_Limit + 5;

% --- BLOCKING CONDITION --------------------------------------
if SOC < Discharge_Limit
    torque_blocked = true;
end

% --- RECOVERY CONDITION --------------------------------------
if torque_blocked
    if SOC >= Recovery_Threshold
        torque_blocked = false;   % SOC recovered enough
    else
        Torque_Out = 0;           % Still blocked
        return
    end
end

% --- NORMAL OPERATION ----------------------------------------
Torque_Out = Torque_In;

end

== matlab function Simulation_Fahrmodell_v4_straight_line_v1/Vehicle Dynamics Model /Drivetrain/Primary and Secondary Axle Powertrain Selector/Primary Axle Powertrain Selector/Hybrid Drive/P0/P0 Motor/SubsysteBattery and Operating Strategy Limitation (Drive)m/Discharge Limit/MATLAB Function ==
  settings: updateMethod=DISCRETE
  data: Torque_In input; SOC input; Torque_Out output; Discharge_Limit input
function Torque_Out = fcn(Torque_In, SOC, Discharge_Limit)

% -------------------------------------------------------------
% Corrected SOC Hysteresis Logic
% -------------------------------------------------------------
% If SOC < Discharge_Limit → torque blocked
% Torque stays blocked until SOC >= Discharge_Limit + 10
% -------------------------------------------------------------

persistent torque_blocked

if isempty(torque_blocked)
    torque_blocked = false;   % Start with torque allowed
end

% Hysteresis threshold
Recovery_Threshold = Discharge_Limit + 5;

% --- BLOCKING CONDITION --------------------------------------
if SOC < Discharge_Limit
    torque_blocked = true;
end

% --- RECOVERY CONDITION --------------------------------------
if torque_blocked
    if SOC >= Recovery_Threshold
        torque_blocked = false;   % SOC recovered enough
    else
        Torque_Out = 0;           % Still blocked
        return
    end
end

% --- NORMAL OPERATION ----------------------------------------
Torque_Out = Torque_In;

end
